simulink model "Final_Power_converter_2018b"  (R2018b)
settings: Solver=VariableStepAuto  StartTime=0.0  StopTime=6  RelTol=1e-3
model workspace (MAT data in the model file):
  Cripple1 = 0.1
  indripple = Simulink.Parameter
  indripple.Value = 0.001
  indripple.DataType = 'auto'
  indripple.DocUnits = 'H'
  indripple.Dimensions = [1 1]
libraries: powerlib x31, simulink x4, powerlib_meascontrol x3
settings Model: OrderedModelArguments=off  Creator=Nicholas  LastModifiedBy=Joseph
settings SolverCC: ZeroCrossAlgorithm=Adaptive
settings DebuggingCC: IgnoredZcDiagnostic=none

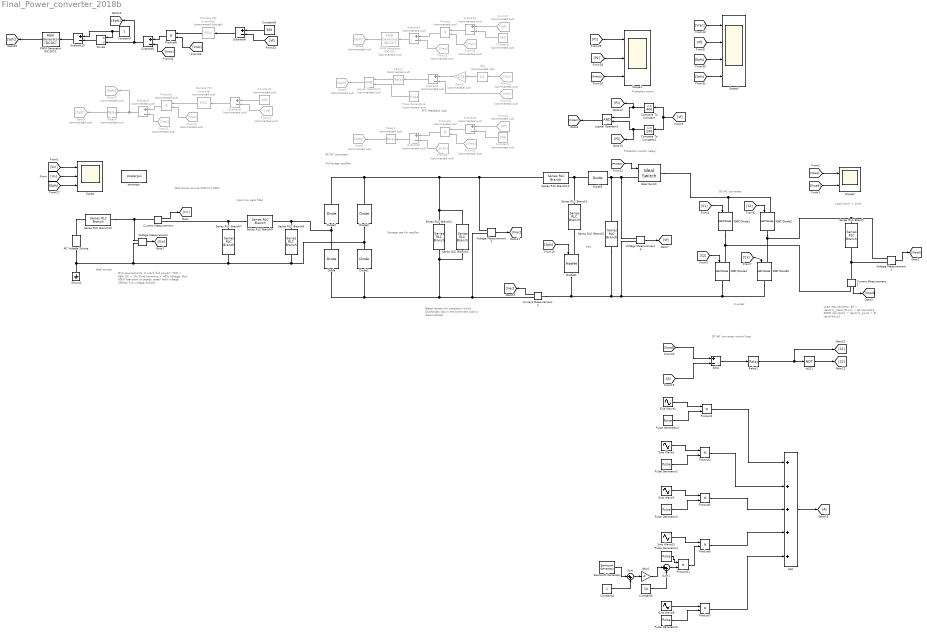
== system Final_Power_converter_2018b ==
  note: Wall power source
      | 220Vrms 50Hz
  note: AC-DC converter
  note: Load
      | 1ohm + 1mH
  note: Load requirements:
      | $0 < \text{I}_{\text{R-L}} < 30 \text{A}$
      | $500\ \text{Hz} < \text{f}_{out} < 5\ \text{kHz}$
  note: Grid requirements:
      | Current (full power):
      | THD < 48%
      | DC < 1%
      | Third harmonic < 40%
      |
      | Voltage:
      | Max 600V (transient or steady state)
      | Hold voltage 200Vdc
      | Trip voltage 400Vdc
  note: DC-AC converter
  note: Full bridge rectifier
  note: Inverter
  note: Ideal source
  note: PFC feedback loop
  note: DC-AC converter control loop
  note: Storage cap for rectifier
  note: Protection switch (relay)
  note: Protection circuit
  note: Bleed resistor for protection circuit.
      | Discharges cap in the event the load is disconnected.
  note: Input low pass filter
  note: PFC
  AC Voltage Source : powerlib/Electrical Sources/AC Voltage Source  Amplitude=220*sqrt(2)  Phase=0  Frequency=50  SampleTime=0  Measurements=None  BusType=PQ  Pref=10e3  Qref=0  Qmin=-inf  Qmax=+inf
      settings: SourceProductName=Simscape Electrical
  Abs : Abs  Commented=on
  Add : Sum  Inputs=5
  Add1 : Sum  Inputs=+-
  Compare To Constant : simulink/Logic and Bit Operations/Compare To Constant  relop=<=  const=400  OutDataTypeStr=boolean
  Compare To Constant1 : simulink/Logic and Bit Operations/Compare To Constant  relop=>=  const=200  OutDataTypeStr=boolean
  Constant1 : Constant  Commented=on  Value=300
  Constant2 : Constant  Commented=on  Value=300
  Constant3 : Constant  Commented=on  Value=300
  Constant4 : Constant
  Constant5 : Constant  Value=10
  Constant6 : Constant  Value=300
  Constant7 : Constant
  Current Measurement : powerlib/Measurements/Current Measurement  PhasorSimulation=off  OutputType=Complex  PSBequivalent=0
      settings: SourceProductName=Simscape Electrical
  Current Measurement1 : powerlib/Measurements/Current Measurement  PhasorSimulation=off  OutputType=Complex  PSBequivalent=0
      settings: SourceProductName=Simscape Electrical
  Current Measurement2 : powerlib/Measurements/Current Measurement  PhasorSimulation=off  OutputType=Complex  PSBequivalent=0
      settings: SourceProductName=Simscape Electrical
  Diode{,1..3} (4 alike) : powerlib/Power Electronics/Diode  Ron=0.001  Lon=0  Vf=1  IC=0  UseSnubber=0  Rs=500  Cs=250e-9  Measurements=off
      settings: SourceProductName=Simscape Electrical
  Diode5 : powerlib/Power Electronics/Diode  Ron=0.001  Lon=0  Vf=0.5  IC=0  UseSnubber=0  Rs=500000  Cs=250e-9  Measurements=off
      settings: SourceProductName=Simscape Electrical
  Discrete PID Controller : simulink/Continuous/PID Controller  Commented=on  Controller=PI  Form=Parallel  TimeDomain=Discrete-time  SampleTime=-1  IntegratorMethod=Forward Euler  FilterMethod=Forward Euler  ControllerParametersSource=internal  P=1  I=2  D=0  UseFilter=on  N=100  TunerSelectOption=Transfer Function Based (PID Tuner App)  InitialConditionSource=internal  InitialConditionForIntegrator=0  InitialConditionForFilter=0  DifferentiatorICPrevScaledInput=0  ExternalReset=none  TrackingMode=off  Kt=1  LimitOutput=off  UpperSaturationLimit=inf  LowerSaturationLimit=-inf  LinearizeAsGain=off  AntiWindupMode=none  Kb=1  POutMin=[]  POutMax=[]  IOutMin=[]  IOutMax=[]  DOutMin=[]  DOutMax=[]  NOutMin=[]  NOutMax=[]  SumOutMin=[]  SumOutMax=[]  SaturationOutMin=[]  SaturationOutMax=[]  PParamMin=[]  PParamMax=[]  IParamMin=[]  IParamMax=[]  DParamMin=[]  DParamMax=[]  NParamMin=[]  NParamMax=[]  KbParamMin=[]  KbParamMax=[]  KtParamMin=[]  KtParamMax=[]  KbOutMin=[]  KbOutMax=[]  KtOutMin=[]  KtOutMax=[]  IntegratorOutMin=[]  IntegratorOutMax=[]  FilterOutMin=[]  FilterOutMax=[]  SumI1OutMin=[]  SumI1OutMax=[]  SumI2OutMin=[]  SumI2OutMax=[]  SumI3OutMin=[]  SumI3OutMax=[]  SumI4OutMin=[]  SumI4OutMax=[]  SumDOutMin=[]  SumDOutMax=[]  DifferentiatorOutMin=[]  DifferentiatorOutMax=[]  FilterDiffOutCoefMin=[]  FilterDiffOutCoefMax=[]  ReciprocalOutMin=[]  ReciprocalOutMax=[]  SumDenOutMin=[]  SumDenOutMax=[]  SumNumOutMin=[]  SumNumOutMax=[]  DivideOutMin=[]  DivideOutMax=[]  IntegratorContinuousStateAttributes=''  IntegratorStateMustResolveToSignalObject=off  IntegratorRTWStateStorageClass=Auto  FilterContinuousStateAttributes=''  FilterStateMustResolveToSignalObject=off  FilterRTWStateStorageClass=Auto  ParallelPVariant=InternalParameters  IdealPVariant=Disabled  IVariant=InternalParameters  DVariant=Disabled  IntegratorVariant=Discrete  SatVariant=Disabled  AWVariant=Passthrough  PCopyVariant=Disabled  TRVariant=Disabled  FdbkBlocksVariant=Forward  IdealPFdbkVariant=Disabled  SatFdbkVariant=Disabled  DerivativeFilterVariant=Disabled  NVariant=Disabled  NCopyVariant=Disabled_SignalSpec  FilterICVariant=Disabled  IntegratorICVariant=InternalICs  ExternalResetVariant=Disabled  TRSumVariant=Passthrough  SumFdbkVariant=Disabled  SumVariant=Sum_PI
  Discrete PID Controller1 : simulink/Continuous/PID Controller  Commented=through  Controller=PI  Form=Parallel  TimeDomain=Discrete-time  SampleTime=-1  IntegratorMethod=Forward Euler  FilterMethod=Forward Euler  ControllerParametersSource=internal  P=1  I=2  D=0  UseFilter=on  N=100  TunerSelectOption=Transfer Function Based (PID Tuner App)  InitialConditionSource=internal  InitialConditionForIntegrator=0  InitialConditionForFilter=0  DifferentiatorICPrevScaledInput=0  ExternalReset=none  TrackingMode=off  Kt=1  LimitOutput=off  UpperSaturationLimit=inf  LowerSaturationLimit=-inf  LinearizeAsGain=off  AntiWindupMode=none  Kb=1  POutMin=[]  POutMax=[]  IOutMin=[]  IOutMax=[]  DOutMin=[]  DOutMax=[]  NOutMin=[]  NOutMax=[]  SumOutMin=[]  SumOutMax=[]  SaturationOutMin=[]  SaturationOutMax=[]  PParamMin=[]  PParamMax=[]  IParamMin=[]  IParamMax=[]  DParamMin=[]  DParamMax=[]  NParamMin=[]  NParamMax=[]  KbParamMin=[]  KbParamMax=[]  KtParamMin=[]  KtParamMax=[]  KbOutMin=[]  KbOutMax=[]  KtOutMin=[]  KtOutMax=[]  IntegratorOutMin=[]  IntegratorOutMax=[]  FilterOutMin=[]  FilterOutMax=[]  SumI1OutMin=[]  SumI1OutMax=[]  SumI2OutMin=[]  SumI2OutMax=[]  SumI3OutMin=[]  SumI3OutMax=[]  SumI4OutMin=[]  SumI4OutMax=[]  SumDOutMin=[]  SumDOutMax=[]  DifferentiatorOutMin=[]  DifferentiatorOutMax=[]  FilterDiffOutCoefMin=[]  FilterDiffOutCoefMax=[]  ReciprocalOutMin=[]  ReciprocalOutMax=[]  SumDenOutMin=[]  SumDenOutMax=[]  SumNumOutMin=[]  SumNumOutMax=[]  DivideOutMin=[]  DivideOutMax=[]  IntegratorContinuousStateAttributes=''  IntegratorStateMustResolveToSignalObject=off  IntegratorRTWStateStorageClass=Auto  FilterContinuousStateAttributes=''  FilterStateMustResolveToSignalObject=off  FilterRTWStateStorageClass=Auto  ParallelPVariant=InternalParameters  IdealPVariant=Disabled  IVariant=InternalParameters  DVariant=Disabled  IntegratorVariant=Discrete  SatVariant=Disabled  AWVariant=Passthrough  PCopyVariant=Disabled  TRVariant=Disabled  FdbkBlocksVariant=Forward  IdealPFdbkVariant=Disabled  SatFdbkVariant=Disabled  DerivativeFilterVariant=Disabled  NVariant=Disabled  NCopyVariant=Disabled_SignalSpec  FilterICVariant=Disabled  IntegratorICVariant=InternalICs  ExternalResetVariant=Disabled  TRSumVariant=Passthrough  SumFdbkVariant=Disabled  SumVariant=Sum_PI
  Divide : Product  Inputs=*/
  From13 : From  Commented=on  GotoTag=Vf
  From14 : From  Commented=on  GotoTag=Vrec
  From{16,21,23,26} (4 alike) : From  Commented=on  GotoTag=Irec
  From17 : From  Commented=on  GotoTag=Vf
  From18 : From  Commented=on  GotoTag=Vrec
  From22 : From  Commented=on  GotoTag=Vin
  From24 : From  Commented=on  GotoTag=Vf
  From25 : From  Commented=on  GotoTag=Vrec
  Gain1 : Gain  Gain=4
  Gain3 : Gain  Commented=on  Gain=0.01
  Goto10 : Goto  Commented=on  GotoTag=Epfc
  Goto{5..6,8..9} (4 alike) : Goto  Commented=on  GotoTag=Spfc
  Ground : powerlib/Elements/Ground  LConnTagsString=a
      settings: SourceProductName=Simscape Electrical
  IGBT/Diode{1..2,4..5} (4 alike) : powerlib/Power Electronics/IGBT//Diode  Ron=1e-3  Rs=10e5  Cs=inf  Measurements=off
      settings: SourceProductName=Simscape Electrical
  Ideal Switch : powerlib/Power Electronics/Ideal Switch  Ron=0.0001  Lon=0  IC=0  Rs=1e6  Cs=inf  Measurements=off
      settings: SourceProductName=Simscape Electrical
  Logical Operator1 : Logic  AllPortsSameDT=off  OutDataTypeStr=boolean
  Logical Operator2 : Logic  Commented=on  AllPortsSameDT=off  OutDataTypeStr=boolean
  Mosfet1 : powerlib/Power Electronics/Mosfet  Ron=0.1  Lon=0  Rd=0.01  Vfd=0  IC=0  Rs=100e6  Cs=inf  Measurements=off
      settings: SourceProductName=Simscape Electrical
  NOT2 : Logic  Operator=NOT  IconShape=distinctive  AllPortsSameDT=off  OutDataTypeStr=boolean
  PWM Generator (DC-DC) : powerlib_meascontrol/Pulse & Signal Generators/PWM Generator (DC-DC)  Commented=on  Fsw=50000  Ts=0
      settings: SourceProductName=Simscape Electrical
  PWM Generator (DC-DC)1 : powerlib_meascontrol/Pulse & Signal Generators/PWM Generator (DC-DC)  Fsw=100000  Ts=0
      settings: SourceProductName=Simscape Electrical
  Product : Product  Commented=on
  Product{1..2,5..8,11} (7 alike) : Product
  Product3 : Product  Commented=on
  Product4 : Product  Commented=on
  Pulse Generator1 : DiscretePulseGenerator  PulseType=Time based  Amplitude=3  Period=6  PulseWidth=1/6*100
  Pulse Generator2 : DiscretePulseGenerator  PulseType=Time based  Amplitude=20  Period=6  PulseWidth=1/3*100  PhaseDelay=1
  Pulse Generator3 : DiscretePulseGenerator  PulseType=Time based  Amplitude=10  Period=6  PulseWidth=1/3*100  PhaseDelay=3
  Pulse Generator4 : DiscretePulseGenerator  PulseType=Time based  Period=6  PulseWidth=1/12*100  PhaseDelay=5
  Pulse Generator5 : DiscretePulseGenerator  PulseType=Time based  Amplitude=18  Period=6  PulseWidth=1/12*100  PhaseDelay=5.5
  Pulse Generator6 : DiscretePulseGenerator  Commented=on  PulseType=Time based  Period=1/50000  PulseWidth=50
  Relay1 : Relay  Commented=on  OnSwitchValue=0.01  OffSwitchValue=-0.01  OnOutputValue=0  OffOutputValue=1
  Relay2 : Relay  OnSwitchValue=0.20  OffSwitchValue=-0.20
  Relay3 : Relay  Commented=on  OnSwitchValue=0.1  OffSwitchValue=-0.1  OnOutputValue=0  OffOutputValue=1
  Relay4 : Relay  Commented=on  OnSwitchValue=3E4  OffSwitchValue=-3E4  OnOutputValue=0  OffOutputValue=1
  Sawtooth Generator : powerlib_meascontrol/Pulse & Signal Generators/Sawtooth Generator  Freq=1/0.5  Phase=0  Ts=0
      settings: SourceProductName=Simscape Electrical
  Scope : Scope  NumInputPorts=3
  Scope1 : Scope  NumInputPorts=3
  Scope2 : Scope  NumInputPorts=2
  Scope3 : Scope  NumInputPorts=4
  Series RLC Branch : powerlib/Elements/Series RLC Branch  LConnTagsString=__new0  RConnTagsString=__new0  BranchType=RL  Resistance=1  Inductance=0.1e-3  SetiL0=off  InitialCurrent=0  Capacitance=1e-6  Setx0=off  InitialVoltage=0  Measurements=None
      settings: SourceProductName=Simscape Electrical
  Series RLC Branch1 : powerlib/Elements/Series RLC Branch  LConnTagsString=__new0  RConnTagsString=__new0  BranchType=L  Resistance=1  Inductance=100e-6  SetiL0=off  InitialCurrent=0  Capacitance=200E-6  Setx0=off  InitialVoltage=0  Measurements=None
      settings: SourceProductName=Simscape Electrical
  Series RLC Branch10 : powerlib/Elements/Series RLC Branch  LConnTagsString=__new0  RConnTagsString=__new0  BranchType=R  Resistance=0.0001  Inductance=160E-9  SetiL0=off  InitialCurrent=0  Capacitance=0.002  Setx0=off  InitialVoltage=0  Measurements=None
      settings: SourceProductName=Simscape Electrical
  Series RLC Branch12 : powerlib/Elements/Series RLC Branch  LConnTagsString=__new0  RConnTagsString=__new0  BranchType=L  Resistance=1  Inductance=100e-6  SetiL0=off  InitialCurrent=0  Capacitance=0.002  Setx0=off  InitialVoltage=0  Measurements=None
      settings: SourceProductName=Simscape Electrical
  Series RLC Branch2 : powerlib/Elements/Series RLC Branch  LConnTagsString=__new0  RConnTagsString=__new0  BranchType=C  Resistance=1  Inductance=0.1e-3  SetiL0=off  InitialCurrent=0  Capacitance=1000E-6  Setx0=off  InitialVoltage=0  Measurements=None
      settings: SourceProductName=Simscape Electrical
  Series RLC Branch3 : powerlib/Elements/Series RLC Branch  LConnTagsString=__new0  RConnTagsString=__new0  BranchType=C  Resistance=1  Inductance=0.1e-3  SetiL0=off  InitialCurrent=0  Capacitance=200E-6  Setx0=off  InitialVoltage=0  Measurements=None
      settings: SourceProductName=Simscape Electrical
  Series RLC Branch4 : powerlib/Elements/Series RLC Branch  LConnTagsString=__new0  RConnTagsString=__new0  BranchType=R  Resistance=2E9  Inductance=0.1e-3  SetiL0=off  InitialCurrent=0  Capacitance=0.001  Setx0=off  InitialVoltage=0  Measurements=None
      settings: SourceProductName=Simscape Electrical
  Series RLC Branch7 : powerlib/Elements/Series RLC Branch  LConnTagsString=__new0  RConnTagsString=__new0  BranchType=C  Resistance=10E9  Inductance=0.1e-3  SetiL0=off  InitialCurrent=0  Capacitance=6.8E-6  Setx0=off  InitialVoltage=0  Measurements=None
      settings: SourceProductName=Simscape Electrical
  Series RLC Branch8 : powerlib/Elements/Series RLC Branch  LConnTagsString=__new0  RConnTagsString=__new0  BranchType=C  Resistance=1  Inductance=0.1e-3  SetiL0=off  InitialCurrent=0  Capacitance=6.8E-6  Setx0=off  InitialVoltage=0  Measurements=None
      settings: SourceProductName=Simscape Electrical
  Series RLC Branch9 : powerlib/Elements/Series RLC Branch  LConnTagsString=__new0  RConnTagsString=__new0  BranchType=L  Resistance=1  Inductance=500E-6  SetiL0=off  InitialCurrent=0  Capacitance=0.002  Setx0=off  InitialVoltage=0  Measurements=None
      settings: SourceProductName=Simscape Electrical
  Sine Wave1 : Sin  Frequency=5000*2*pi  SampleTime=0
  Sine Wave10 : Sin  Frequency=1000*2*pi  SampleTime=0
  Sine Wave5 : Sin  Frequency=500*2*pi  SampleTime=0
  Sine Wave7 : Sin  Frequency=1000*2*pi  SampleTime=0
  Sine Wave8 : Sin  Frequency=1000*2*pi  SampleTime=0
  Subtract{1..7} (7 alike) : Sum  Commented=on  Inputs=+-
  Subtract10 : Sum  Inputs=+-
  Subtract8 : Sum  Inputs=+-
  Subtract9 : Sum  Inputs=+-
  Sum : Sum  Inputs=|++
  Sum1 : Sum  Inputs=|++
  Voltage Measurement{,1,3..4} (4 alike) : powerlib/Measurements/Voltage Measurement  PhasorSimulation=off  OutputType=Complex  PSBequivalent=0
      settings: SourceProductName=Simscape Electrical
  powergui : powerlib/powergui  Priority=1  SimulationMode=Discrete  SampleTime=1E-6  frequency=60  Iterations=50  frequencyindice=0  Pbase=100e6  ErrMax=1e-4  UnitsV=kV  UnitsW=MW  buscounter=0  FunctionMessages=off  echomessages=off  EnableUseOfTLC=off  CurrentSourceSwitches=off  DisableSnubberDevices=off  DisableRonSwitches=off  DisableVfSwitches=off  DisplayEquations=off  SolverType=Tustin/Backward Euler (TBE)  Interpol=off  ExternalGateDelay=off  methode=off  Ts=100  x0status=blocks  SPID=on  SwTol=0  HookPort=off  RestoreLinks=warning  ResistiveCurrentMeasurement=off  Frange=[0:2:500]  Ylog=off  Xlog=on  ShowGrid=off  save=off  variable=ZData  structure=ScopeData  ZoomFFT=on  StartTime=1  cycles=1  DisplayStyle=2  fundamental=50  FreqAxis=off  MaxFrequency=2000  frequencyindicesteady=1  RmsSteady=1  display=off
      settings: SourceProductName=Simscape Electrical
  wires:
  Voltage Measurement/1 -> [Vin]
  Current Measurement/1 -> [Iin]
  Voltage Measurement1/1 -> [Vload]
  [Iin] -> Scope/2
  [Vin] -> Scope/1
  Current Measurement1/1 -> [Iload]
  [S2] -> IGBT/Diode2/1
  [S2] -> IGBT/Diode4/1
  [S1] -> IGBT/Diode1/1
  [S1] -> IGBT/Diode5/1
  [Vload] -> Scope2/1
  [Iload] -> Scope2/2
  Voltage Measurement3/1 -> [Vrec]
  [Vrec] -> Scope3/1
  Current Measurement2/1 -> [Irec]
  [Iload] -> Add1/1
  Sine Wave5/1 -> Product1/1
  Sum1/1 -> Product11/2
  Constant5/1 -> Sum1/2
  Add1/1 -> Relay2/1
  Product1/1 -> Add/1
  Product11/1 -> Product6/2
  Gain1/1 -> Sum1/1
  Constant4/1 -> Sum/2
  [A] -> Add1/2
  Sawtooth Generator/1 -> Sum/1
  Product5/1 -> Add/3
  Add/1 -> [A]
  Sine Wave1/1 -> Product2/1
  Product7/1 -> Add/5
  Pulse Generator2/1 -> Product2/2
  Sum/1 -> Gain1/1
  Product6/1 -> Add/4
  Sine Wave8/1 -> Product7/1
  Product2/1 -> Add/2
  Pulse Generator3/1 -> Product5/2
  Sine Wave10/1 -> Product6/1
  Pulse Generator4/1 -> Product11/1
  Pulse Generator1/1 -> Product1/2
  Sine Wave7/1 -> Product5/1
  Pulse Generator5/1 -> Product7/2
  NOT2/1 -> [S2]
  From16/1 -> Subtract2/2
  Gain3/1 -> Subtract2/1
  Abs/1 -> Gain3/1
  From22/1 -> Abs/1
  Subtract2/1 -> Relay1/1
  Compare To Constant1/1 -> [P2], Logical Operator1/2
  [Protect] -> Ideal Switch/1
  Compare To Constant/1 -> Logical Operator1/1, [P1]
  [Vf] -> Compare To Constant/1, Compare To Constant1/1
  Logical Operator1/1 -> [Protect]
  [Spfc] -> Mosfet1/1
  Pulse Generator6/1 -> Logical Operator2/2
  Relay1/1 -> Logical Operator2/1
  Logical Operator2/1 -> Goto5/1
  Relay2/1 -> NOT2/1, [S1]
  Voltage Measurement4/1 -> [Vf]
  Constant1/1 -> Subtract1/2
  From17/1 -> Subtract1/1
  Subtract1/1 -> Product/1
  From18/1 -> Product/2
  Product/1 -> Subtract3/1
  From23/1 -> Subtract3/2
  Subtract3/1 -> PWM Generator (DC-DC)/1
  PWM Generator (DC-DC)/1 -> Goto8/1
  Constant2/1 -> Subtract4/2
  Subtract5/1 -> Relay3/1
  Subtract4/1 -> Product3/1
  Relay3/1 -> Goto6/1
  From25/1 -> Product3/2
  From26/1 -> Subtract5/2
  From24/1 -> Subtract4/1
  Product3/1 -> Subtract5/1
  [Vf] -> Scope3/2
  Product4/1 -> Subtract7/1
  Subtract7/1 -> Goto10/1, Relay4/1
  From13/1 -> Subtract6/2
  Relay4/1 -> Goto9/1
  From21/1 -> Subtract7/2
  From14/1 -> Product4/2
  Constant3/1 -> Subtract6/1
  Subtract6/1 -> Discrete PID Controller/1
  Discrete PID Controller/1 -> Product4/1
  [Epfc] -> Scope/3
  [Protect] -> Scope1/3
  [P1] -> Scope1/1
  [P2] -> Scope1/2
  [Epfc] -> Scope3/3
  [Spfc] -> Scope3/4
  Product8/1 -> Subtract9/1
  [Irec] -> Subtract9/2
  Discrete PID Controller1/1 -> Product8/1
  PWM Generator (DC-DC)1/1 -> [Spfc]
  Subtract8/1 -> Discrete PID Controller1/1
  [Vrec] -> Product8/2
  [Vf] -> Subtract8/2
  Subtract9/1 -> Divide/2, [Epfc]
  Constant6/1 -> Subtract8/1
  Constant7/1 -> Subtract10/1, Divide/1
  Divide/1 -> Subtract10/2
  Subtract10/1 -> PWM Generator (DC-DC)1/1
  connections:
  Voltage Measurement/LConn1 -- Series RLC Branch10/RConn1 -- Current Measurement/LConn1
  Current Measurement1/LConn1 -- Voltage Measurement1/LConn2 -- Series RLC Branch/RConn1
  Series RLC Branch2/RConn1 -- Mosfet1/RConn1 -- Current Measurement2/LConn1 -- Voltage Measurement4/LConn2 -- IGBT/Diode4/RConn1 -- IGBT/Diode5/RConn1
  IGBT/Diode1/RConn1 -- Current Measurement1/RConn1 -- IGBT/Diode4/LConn1
  Series RLC Branch10/LConn1 -- AC Voltage Source/RConn1
  IGBT/Diode2/RConn1 -- Voltage Measurement1/LConn1 -- Series RLC Branch/LConn1 -- IGBT/Diode5/LConn1
  Series RLC Branch7/LConn1 -- Current Measurement/RConn1 -- Series RLC Branch9/LConn1
  Diode/LConn1 -- Voltage Measurement3/LConn2 -- Current Measurement2/RConn1 -- Series RLC Branch4/RConn1 -- Series RLC Branch3/RConn1 -- Diode1/LConn1
  AC Voltage Source/LConn1 -- Ground/LConn1 -- Voltage Measurement/LConn2 -- Diode3/LConn1 -- Diode1/RConn1 -- Series RLC Branch8/RConn1 -- Series RLC Branch7/RConn1
  Diode2/RConn1 -- Series RLC Branch4/LConn1 -- Series RLC Branch3/LConn1 -- Series RLC Branch12/LConn1 -- Voltage Measurement3/LConn1 -- Diode3/RConn1
  Series RLC Branch8/LConn1 -- Diode2/LConn1 -- Diode/RConn1 -- Series RLC Branch9/RConn1
  IGBT/Diode1/LConn1 -- Ideal Switch/RConn1 -- IGBT/Diode2/LConn1
  Series RLC Branch1/LConn1 -- Series RLC Branch12/RConn1 -- Diode5/LConn1
  Series RLC Branch1/RConn1 -- Mosfet1/LConn1
  Ideal Switch/LConn1 -- Series RLC Branch2/LConn1 -- Diode5/RConn1 -- Voltage Measurement4/LConn1
